simulink model "emerging_simulink_model"  (R2019a)
settings: Solver=VariableStepAuto  StartTime=0.0  StopTime=15  RelTol=1e-3
libraries: mpclib x1, simulink x1
settings Model: Creator=alexh  LastModifiedBy=alexh

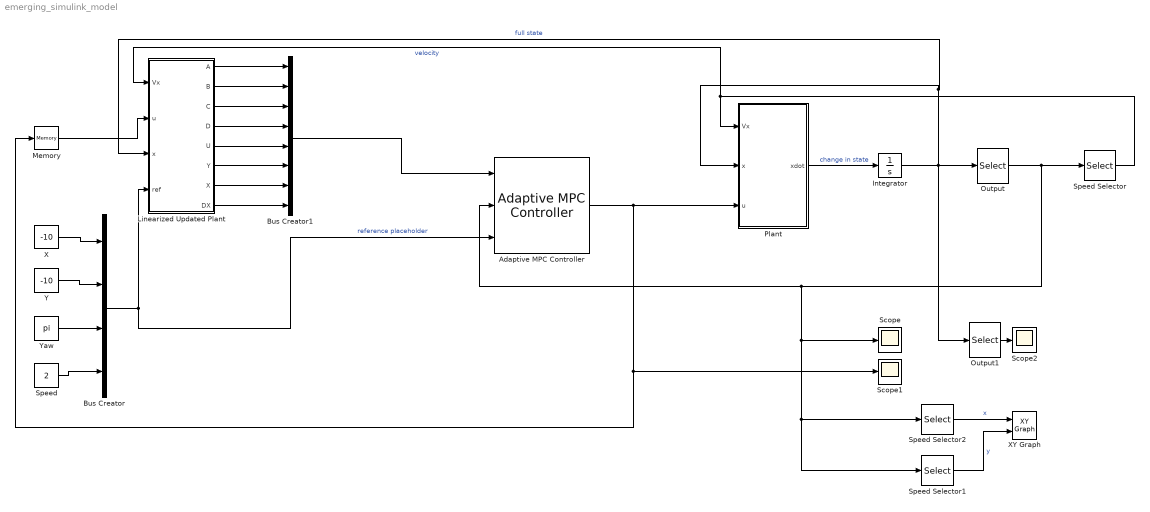
== system emerging_simulink_model ==
  Adaptive MPC Controller : mpclib/Adaptive MPC Controller  SCDEnableBlockLinearizationSpecification=on  mpcobj=bycicle_mpc  enable_value=0  updateMPCinCallerWorkspace=on  md_inport=off  mv_inport=off  uref_inport=off  return_cost=off  return_mvseq=off  return_qpstatus=off  return_xseq=off  return_state=off  return_ovseq=off  state_inport=off  isltv_plant=off  umin_inport=off  umax_inport=off  ymin_inport=off  ymax_inport=off  cc_inport=off  ywt_inport=off  uwt_inport=off  duwt_inport=off  rhoeps_inport=off  pm_inport=off  MaximumP=10  HorizonChoice=FixedHorizon  BlockDataType=double  SampleTimeInherited=off  switch_inport=off
      settings: SourceProductName=MATLAB Runtime - Model Predictive Control Toolbox Addin  SourceProductBaseCode=Missing
  Bus Creator : BusCreator  Inputs=4
  Bus Creator1 : BusCreator  Inputs=8
  Integrator : Integrator
  Linearized Updated Plant : MATLAB Function  TreatAsAtomicUnit=on
  Memory : Memory
  Output : Selector  InputPortWidth=6  IndexOptions=Index vector (dialog)  Indices=[1, 2, 3, 6]  OutputSizes=1
  Output1 : Selector  InputPortWidth=6  IndexOptions=Index vector (dialog)  Indices=[4, 5]  OutputSizes=1
  "Plant " : MATLAB Function  TreatAsAtomicUnit=on
  Scope : Scope
  Scope1 : Scope
  Scope2 : Scope
  Speed : Constant  Value=2
  Speed Selector : Selector  InputPortWidth=4  IndexOptions=Index vector (dialog)  Indices=[4]  OutputSizes=1
  Speed Selector1 : Selector  InputPortWidth=4  IndexOptions=Index vector (dialog)  Indices=[2]  OutputSizes=1
  Speed Selector2 : Selector  InputPortWidth=4  IndexOptions=Index vector (dialog)  Indices=[1]  OutputSizes=1
  X : Constant  Value=-10
  XY Graph : simulink/Sinks/XY Graph  xmin=-15  xmax=15  ymin=-15  ymax=15  st=-1
  Y : Constant  Value=-10
  Yaw : Constant  Value=pi
  wires:
  Adaptive MPC Controller/1 -> Scope1/1, Memory/1, "Plant "/3(u)
  "Plant "/1(xdot) -> Integrator/1  "change in state"
  Integrator/1 -> Output1/1, Linearized Updated Plant/3(x), "Plant "/2(x), Output/1  "full state"
  Output/1 -> Speed Selector1/1, Speed Selector2/1, Scope/1, Adaptive MPC Controller/2, Speed Selector/1
  Y/1 -> Bus Creator/2
  Yaw/1 -> Bus Creator/3
  Speed/1 -> Bus Creator/4
  Bus Creator/1 -> Adaptive MPC Controller/3, Linearized Updated Plant/4(ref)  "reference placeholder"
  Linearized Updated Plant/1(A) -> Bus Creator1/1
  Linearized Updated Plant/2(B) -> Bus Creator1/2
  Linearized Updated Plant/3(C) -> Bus Creator1/3
  Linearized Updated Plant/4(D) -> Bus Creator1/4
  Linearized Updated Plant/5(U) -> Bus Creator1/5
  Linearized Updated Plant/6(Y) -> Bus Creator1/6
  Linearized Updated Plant/7(X) -> Bus Creator1/7
  Linearized Updated Plant/8(DX) -> Bus Creator1/8
  Bus Creator1/1 -> Adaptive MPC Controller/1
  Memory/1 -> Linearized Updated Plant/2(u)
  Speed Selector/1 -> Linearized Updated Plant/1(Vx), "Plant "/1(Vx)  "velocity"
  X/1 -> Bus Creator/1
  Output1/1 -> Scope2/1
  Speed Selector1/1 -> XY Graph/2  "y"
  Speed Selector2/1 -> XY Graph/1  "x"

== matlab function emerging_simulink_model/Linearized Updated Plant ==
  data: Vx input; u input; A output; x input; B output; C output; D output; U output; Y output; X output; DX output; ref input
function [A,B,C,D,U,Y,X,DX] = fcn(Vx,u,x, ref)
% Sample time
Ts = 0.1;

% Model parameters
m = 1575;
iz = 2875;
lf = 1.2;
lr = 1.6;
cf = 19000;
cr = 33000;

if (Vx<0.5)
       Vx = 0.5;
end

% we have to tweak the system a bit to make it realize altering the 
% speed can do something for reaching the destination
if (x(2)<ref(2))
    speed_influence = 0.1;
else
    speed_influence = -0.1;
end

% Continuous-time model
Ac = [0, 0, -Vx, 0, -1, Vx;
       0, 0, Vx, 0, 1, speed_influence;
       0, 0, 0, 1, 0, 0;
       0, 0, 0, -(2*cf*lf^2+2*cr*lr^2)/iz/Vx, -(2*cf*lf-2*cr*lr)/iz/Vx, 0;
       0, 0, 0,  -Vx-(2*cf*lf-2*cr*lr)/m/Vx, -(2*cf+2*cr)/m/Vx, 0;
       0, 0, 0, 0, 0, -.1];
   
 Bc = [0, 0, 0, 2*cf*lf/iz, 2*cf/m, 0;
        0, 0, 0, 0, 0, 1]';
 
 % Position, Yaw, Speed
 Cc = [1, 0, 0, 0, 0, 0;
        0, 1, 0, 0, 0, 0;
        0, 0, 1, 0, 0, 0;
        0, 0, 0, 0, 0, 1];
    
 Dc = zeros(4, 2);

% Generate discrete-time model
nx = size(Ac,1);
nu = size(Bc,2);
M = expm([[Ac Bc]*Ts; zeros(nu,nx+nu)]);
A = M(1:nx,1:nx);
B = M(1:nx,nx+1:nx+nu);
C = Cc;
D = Dc;

% Nominal conditions for discrete-time plant
X = x';
U = u';
Y = (C*x + D*u)';
DX = (A*x+B*u-x)';      % did this fix, might be wrong

== matlab function emerging_simulink_model/Plant  ==
  data: Vx input; x input; u input; xdot output
function xdot = fcn(Vx,x,u)

if (Vx<0.01)
    Vx=0.01;
end

% Model parameters
m = 1575;
iz = 2875;
lf = 1.2;
lr = 1.6;
cf = 19000;
cr = 33000;

sin_yaw = sin(x(3));
cos_yaw = cos(x(3));


% Continuous-time model
% Continuous-time model
Ac = [0, 0, 0, 0, 0, cos_yaw;
       0, 0, 0, 0, 0, sin_yaw;
       0, 0, 0, 1, 0, 0;
       0, 0, 0, -(2*cf*lf^2+2*cr*lr^2)/iz/Vx, -(2*cf*lf-2*cr*lr)/iz/Vx, 0;
       0, 0, 0,  -Vx-(2*cf*lf-2*cr*lr)/m/Vx, -(2*cf+2*cr)/m/Vx, 0;
       0, 0, 0, 0, 0, -.1];
   
 Bc = [0, 0, 0, 2*cf*lf/iz, 2*cf/m, 0;
        0, 0, 0, 0, 0, 1]';

xdot = Ac*x + Bc*u;
